simulink model "CDCJournalModel"  (R2017a)
settings: Solver=FixedStepAuto  StartTime=0.0  StopTime=p.T  FixedStep=0.001  RelTol=1e-3
StopFcn:
  | stopCallback
values from neighbouring files (symbols this model uses):
  p = simulationParametersClass    [preLoadCallback.m]
undefined symbols (not defined in the file or in its folder): rudderTable, wingTable
libraries: simulink x9, myLibrary x9, lowLevel x6, dspsigops x1
settings Model: Creator=M.Cobb  LastModifiedBy=M.Cobb
settings DataIOCC: SaveFormat=Structure

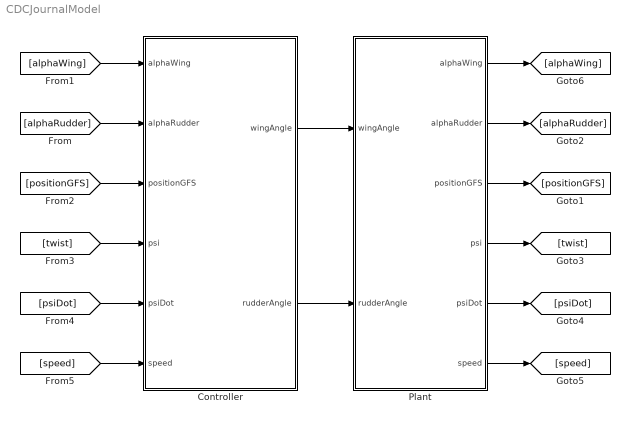
== system CDCJournalModel ==
  Controller : Subsystem
  Plant : Subsystem
  wires:
  Controller/1(wingAngle) -> Plant/1(wingAngle)
  Plant/1(alphaWing) -> [alphaWing]
  Plant/2(alphaRudder) -> [alphaRudder]
  [alphaWing] -> Controller/1(alphaWing)
  [alphaRudder] -> Controller/2(alphaRudder)
  Plant/3(positionGFS) -> [positionGFS]
  [positionGFS] -> Controller/3(positionGFS)
  Plant/4(psi) -> [twist]
  [twist] -> Controller/4("psi ")
  [psiDot] -> Controller/5(psiDot)
  [speed] -> Controller/6(speed)
  Plant/5(psiDot) -> [psiDot]
  Plant/6(speed) -> [speed]
  Controller/2(rudderAngle) -> Plant/2(rudderAngle)

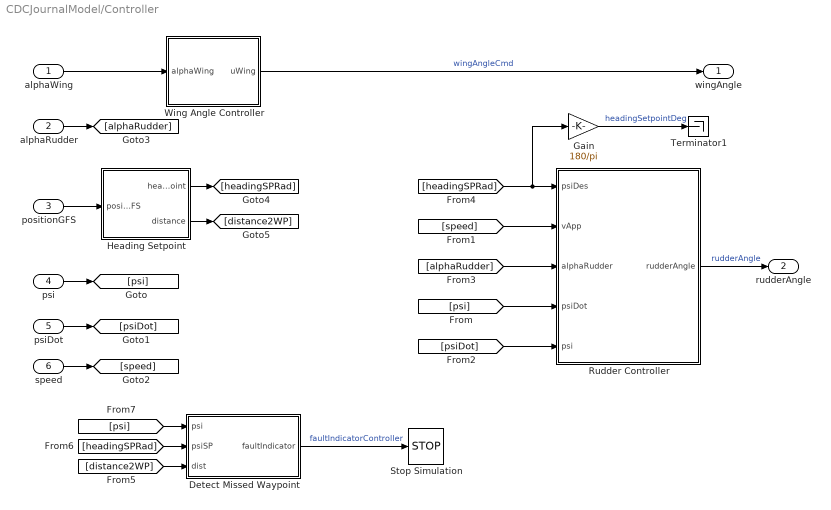
== system CDCJournalModel/Controller ==
  alphaWing : Inport
  alphaRudder : Inport  Port=2
  positionGFS : Inport  Port=3
  "psi " : Inport  Port=4
  psiDot : Inport  Port=5
  speed : Inport  Port=6
  Detect Missed Waypoint : Subsystem
  Gain : Gain  Gain=180/pi
  Heading Setpoint : Subsystem
  Rudder Controller : Subsystem
  Stop Simulation : Stop
  Terminator1 : Terminator
  Wing Angle Controller : Subsystem
  wingAngle : Outport
  rudderAngle : Outport  Port=2
  wires:
  alphaWing/1 -> Wing Angle Controller/1(alphaWing)
  Wing Angle Controller/1(uWing) -> wingAngle/1  "wingAngleCmd"
  positionGFS/1 -> Heading Setpoint/1(positionGFS)
  Heading Setpoint/1(headingSetpoint) -> [headingSPRad]
  "psi "/1 -> [psi]
  psiDot/1 -> [psiDot]
  speed/1 -> [speed]
  alphaRudder/1 -> [alphaRudder]
  Gain/1 -> Terminator1/1  "headingSetpointDeg"
  Rudder Controller/1(rudderAngle) -> rudderAngle/1  "rudderAngle"
  [speed] -> Rudder Controller/2(vApp)
  [headingSPRad] -> Gain/1, Rudder Controller/1(psiDes)
  [alphaRudder] -> Rudder Controller/3(alphaRudder)
  [psi] -> Rudder Controller/4(psiDot)
  [psiDot] -> Rudder Controller/5(psi)
  Heading Setpoint/2(distance) -> [distance2WP]
  [distance2WP] -> Detect Missed Waypoint/3("dist ")
  [psi] -> Detect Missed Waypoint/1(psi)
  [headingSPRad] -> Detect Missed Waypoint/2(psiSP)
  Detect Missed Waypoint/1(faultIndicator) -> Stop Simulation/1  "faultIndicatorController"

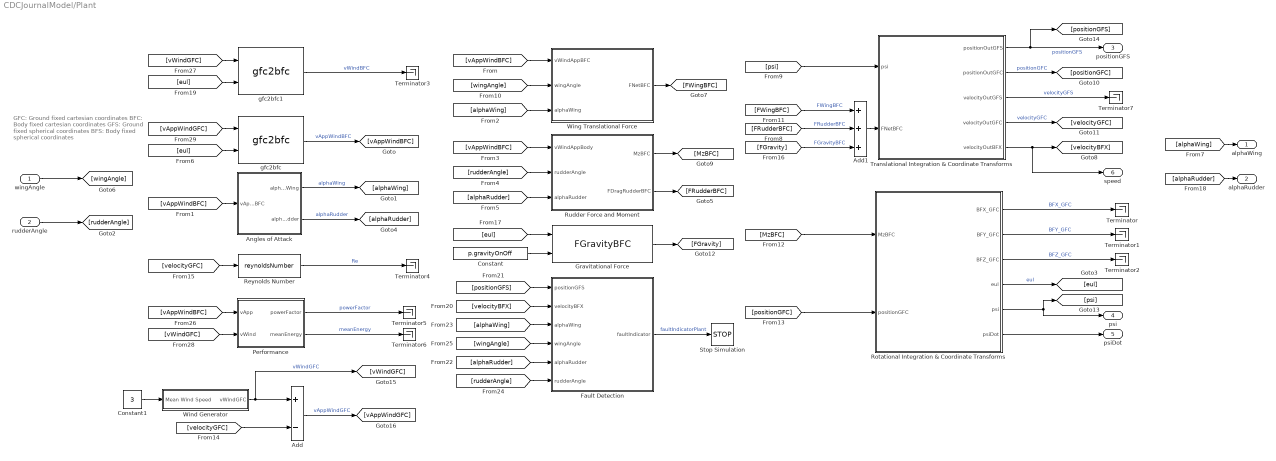
== system CDCJournalModel/Plant ==
  note: GFC: Ground fixed cartesian coordinates
      | BFC:  Body fixed cartesian coordinates
      | GFS: Ground fixed spherical coordinates
      | BFS: Body fixed spherical coordinates
  wingAngle : Inport
  rudderAngle : Inport  Port=2
  Add : Sum  Inputs=+-
  Add1 : Sum  Inputs=+++
  Angles of Attack : Subsystem
  Constant : Constant  Value=p.gravityOnOff
  Constant1 : Constant  Value=3
  Fault Detection : Subsystem
  Gravitational Force : myLibrary/FGravityBFC
  Performance : Subsystem
  Reynolds Number : myLibrary/reynoldsNumber
  Rotational Integration & Coordinate Transforms : Subsystem
  Rudder Force and Moment : Subsystem
  Stop Simulation : Stop
  Terminator{,1..7} (8 alike) : Terminator
  Translational Integration & Coordinate Transforms : Subsystem
  Wind Generator : Subsystem
  Wing Translational Force : Subsystem
  gfc2bfc : myLibrary/gfc2bfc
  gfc2bfc1 : myLibrary/gfc2bfc
  alphaWing : Outport
  alphaRudder : Outport  Port=2
  positionGFS : Outport  Port=3
  psi : Outport  Port=4
  psiDot : Outport  Port=5
  speed : Outport  Port=6
  wires:
  Wind Generator/1(vWindGFC) -> [vWindGFC], Add/1  "vWindGFC"
  [vAppWindBFC] -> Angles of Attack/1(vAppWindBFC)
  Angles of Attack/1(alphaWing) -> [alphaWing]  "alphaWing"
  [vAppWindBFC] -> Wing Translational Force/1(vWindAppBFC)
  Add/1 -> [vAppWindGFC]  "vAppWindGFC"
  [vAppWindBFC] -> Rudder Force and Moment/1(vWindAppBody)
  rudderAngle/1 -> [rudderAngle]
  [rudderAngle] -> Rudder Force and Moment/2(rudderAngle)
  Translational Integration & Coordinate Transforms/2(positionOutGFC) -> [positionGFC]  "positionGFC"
  Rudder Force and Moment/2(FDragRudderBFC) -> [FRudderBFC]
  [alphaWing] -> Wing Translational Force/3(alphaWing)
  [psi] -> Translational Integration & Coordinate Transforms/1(psi)
  Angles of Attack/2(alphaRudder) -> [alphaRudder]  "alphaRudder"
  [alphaRudder] -> Rudder Force and Moment/3(alphaRudder)
  wingAngle/1 -> [wingAngle]
  [FRudderBFC] -> Add1/2  "FRudderBFC"
  Wing Translational Force/1(FNetBFC) -> [FWingBFC]
  [wingAngle] -> Wing Translational Force/2(wingAngle)
  Add1/1 -> Translational Integration & Coordinate Transforms/2(FNetBFC)
  [FWingBFC] -> Add1/1  "FWingBFC"
  Rudder Force and Moment/1(MzBFC) -> [MzBFC]
  [MzBFC] -> Rotational Integration & Coordinate Transforms/1(MzBFC)
  [positionGFC] -> Rotational Integration & Coordinate Transforms/2(positionGFC)
  Rotational Integration & Coordinate Transforms/4(eul) -> [eul]  "eul"
  Rotational Integration & Coordinate Transforms/1(BFX_GFC) -> Terminator/1  "BFX_GFC"
  Rotational Integration & Coordinate Transforms/2(BFY_GFC) -> Terminator1/1  "BFY_GFC"
  Rotational Integration & Coordinate Transforms/3(BFZ_GFC) -> Terminator2/1  "BFZ_GFC"
  Translational Integration & Coordinate Transforms/4(velocityOutGFC) -> [velocityGFC]  "velocityGFC"
  [velocityGFC] -> Add/2
  [velocityGFC] -> Reynolds Number/1
  Reynolds Number/1 -> Terminator4/1  "Re"
  [FGravity] -> Add1/3  "FGravityBFC"
  Gravitational Force/1 -> [FGravity]
  [eul] -> Gravitational Force/1
  Translational Integration & Coordinate Transforms/1(positionOutGFS) -> positionGFS/1, [positionGFS]  "positionGFS"
  Translational Integration & Coordinate Transforms/3(velocityOutGFS) -> Terminator7/1  "velocityGFS"
  [eul] -> gfc2bfc1/2
  gfc2bfc1/1 -> Terminator3/1  "vWindBFC"
  Rotational Integration & Coordinate Transforms/5(psi) -> [psi], psi/1
  Constant/1 -> Gravitational Force/2
  [alphaWing] -> alphaWing/1
  [alphaRudder] -> alphaRudder/1
  Constant1/1 -> Wind Generator/1(Mean Wind Speed)
  Translational Integration & Coordinate Transforms/5(velocityOutBFX) -> speed/1, [velocityBFX]
  [velocityBFX] -> Fault Detection/2(velocityBFX)
  [positionGFS] -> Fault Detection/1(positionGFS)
  Fault Detection/1(faultIndicator) -> Stop Simulation/1  "faultIndicatorPlant"
  [alphaRudder] -> Fault Detection/5(alphaRudder)
  [alphaWing] -> Fault Detection/3(alphaWing)
  [rudderAngle] -> Fault Detection/6(rudderAngle)
  [wingAngle] -> Fault Detection/4(wingAngle)
  Rotational Integration & Coordinate Transforms/6(psiDot) -> psiDot/1
  [vWindGFC] -> gfc2bfc1/1
  [vAppWindBFC] -> Performance/1(vApp)
  [vWindGFC] -> Performance/2(vWind)
  gfc2bfc/1 -> [vAppWindBFC]  "vAppWindBFC"
  [eul] -> gfc2bfc/2
  [vAppWindGFC] -> gfc2bfc/1
  Performance/1(powerFactor) -> Terminator5/1  "powerFactor"
  Performance/2(meanEnergy) -> Terminator6/1  "meanEnergy"

== system CDCJournalModel/Controller/Detect Missed Waypoint ==
  psi : Inport
  psiSP : Inport  Port=2
  "dist " : Inport  Port=3
  Abs : Abs
  Add : Sum  Inputs=+-
  Add1 : Sum  Inputs=-+
  Compare To Constant : simulink/Logic and Bit Operations/Compare To Constant  relop=>=  const=pi/2  OutDataTypeStr=boolean
  Compare To Constant1 : simulink/Logic and Bit Operations/Compare To Constant  relop=<  const=0  OutDataTypeStr=boolean
  Delay : Delay  DelayLength=1  InitialCondition=0
  Logical Operator : Logic  AllPortsSameDT=off  OutDataTypeStr=boolean
  faultIndicator : Outport
  wires:
  Compare To Constant/1 -> Logical Operator/1
  psiSP/1 -> Add/1
  Delay/1 -> Add1/2
  Add1/1 -> Compare To Constant1/1
  Add/1 -> Abs/1
  psi/1 -> Add/2
  Logical Operator/1 -> faultIndicator/1  "faultMissedWaypoint"
  Compare To Constant1/1 -> Logical Operator/2
  Abs/1 -> Compare To Constant/1
  "dist "/1 -> Delay/1, Add1/1

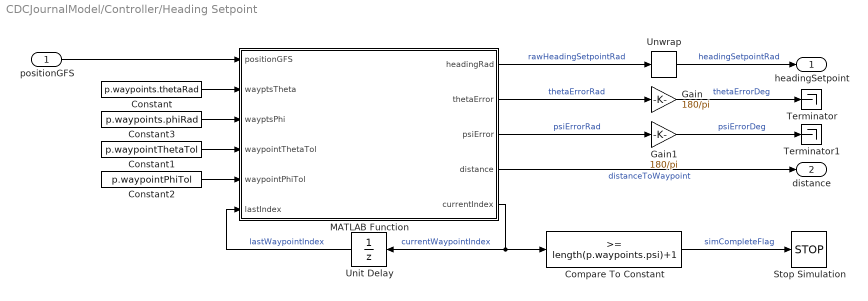
== system CDCJournalModel/Controller/Heading Setpoint ==
  positionGFS : Inport
  Compare To Constant : simulink/Logic and Bit Operations/Compare To Constant  relop=>=  const=length(p.waypoints.psi)+1  OutDataTypeStr=boolean
  Constant : Constant  Value=p.waypoints.thetaRad
  Constant1 : Constant  Value=p.waypointThetaTol
  Constant2 : Constant  Value=p.waypointPhiTol
  Constant3 : Constant  Value=p.waypoints.phiRad
  Gain : Gain  Gain=180/pi
  Gain1 : Gain  Gain=180/pi
  MATLAB Function : MATLAB Function  TreatAsAtomicUnit=on
  Stop Simulation : Stop
  Terminator : Terminator
  Terminator1 : Terminator
  Unit Delay : UnitDelay  InitialCondition=1  SampleTime=-1
  Unwrap : dspsigops/Unwrap  tol=pi  InputProcessing=Columns as channels (frame based)  running=off
  headingSetpoint : Outport
  distance : Outport  Port=2
  wires:
  Constant1/1 -> MATLAB Function/4(waypointThetaTol)
  Unit Delay/1 -> MATLAB Function/6(lastIndex)  "lastWaypointIndex"
  Constant2/1 -> MATLAB Function/5(waypointPhiTol)
  positionGFS/1 -> MATLAB Function/1(positionGFS)
  Constant/1 -> MATLAB Function/2(wayptsTheta)
  Constant3/1 -> MATLAB Function/3(wayptsPhi)
  MATLAB Function/2(thetaError) -> Gain/1  "thetaErrorRad"
  MATLAB Function/3(psiError) -> Gain1/1  "psiErrorRad"
  Gain/1 -> Terminator/1  "thetaErrorDeg"
  Gain1/1 -> Terminator1/1  "psiErrorDeg"
  MATLAB Function/5(currentIndex) -> Compare To Constant/1, Unit Delay/1  "currentWaypointIndex"
  MATLAB Function/1(headingRad) -> Unwrap/1  "rawHeadingSetpointRad"
  Unwrap/1 -> headingSetpoint/1  "headingSetpointRad"
  Compare To Constant/1 -> Stop Simulation/1  "simCompleteFlag"
  MATLAB Function/4(distance) -> distance/1  "distanceToWaypoint"

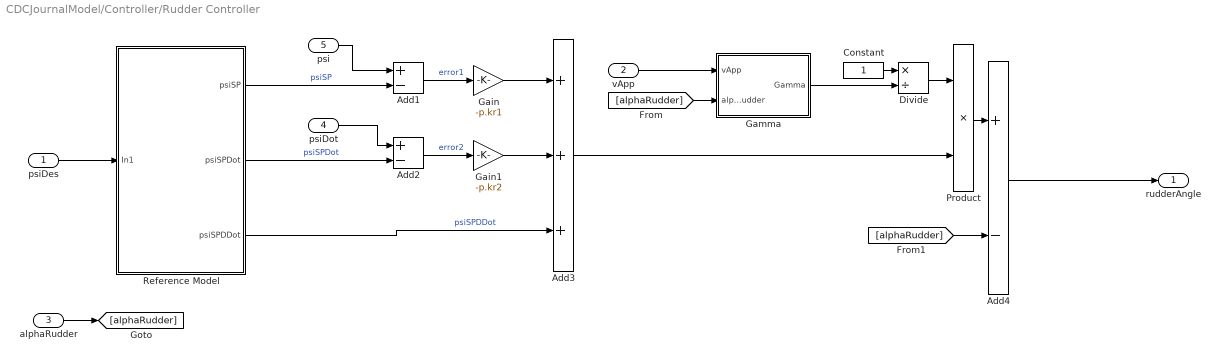
== system CDCJournalModel/Controller/Rudder Controller ==
  psiDes : Inport
  vApp : Inport  Port=2
  alphaRudder : Inport  Port=3
  psiDot : Inport  Port=4
  psi : Inport  Port=5
  Add1 : Sum  Inputs=+-
  Add2 : Sum  Inputs=+-
  Add3 : Sum  Inputs=+++
  Add4 : Sum  Inputs=+-
  Constant : Constant
  Divide : Product  Inputs=*/
  Gain : Gain  Gain=-p.kr1
  Gain1 : Gain  Gain=-p.kr2
  Gamma : Subsystem
  Product : Product
  Reference Model : Subsystem
  rudderAngle : Outport
  wires:
  alphaRudder/1 -> [alphaRudder]
  vApp/1 -> Gamma/1(vApp)
  [alphaRudder] -> Gamma/2(alphaRudder)
  [alphaRudder] -> Add4/2
  Product/1 -> Add4/1
  Gamma/1(Gamma) -> Divide/2
  Divide/1 -> Product/1
  Constant/1 -> Divide/1
  Add2/1 -> Gain1/1  "error2"
  Add1/1 -> Gain/1  "error1"
  Reference Model/1(psiSP) -> Add1/2  "psiSP"
  Reference Model/2(psiSPDot) -> Add2/2  "psiSPDot"
  psi/1 -> Add1/1
  Gain1/1 -> Add3/2
  psiDot/1 -> Add2/1
  Reference Model/3(psiSPDDot) -> Add3/3  "psiSPDDot"
  Gain/1 -> Add3/1
  psiDes/1 -> Reference Model/1(In1)
  Add3/1 -> Product/2
  Add4/1 -> rudderAngle/1

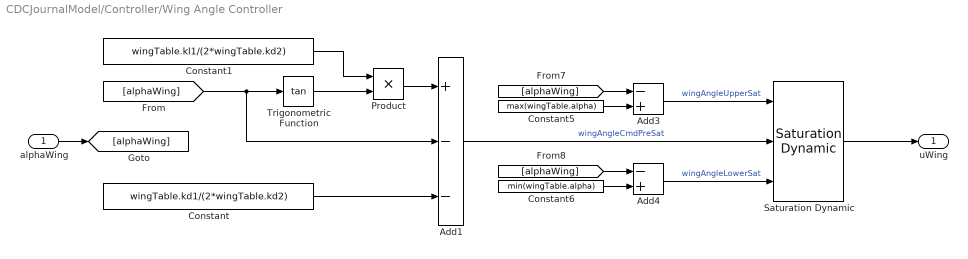
== system CDCJournalModel/Controller/Wing Angle Controller ==
  alphaWing : Inport
  Add1 : Sum  Inputs=+--
  Add3 : Sum  Inputs=-+
  Add4 : Sum  Inputs=-+
  Constant : Constant  Value=wingTable.kd1/(2*wingTable.kd2)
  Constant1 : Constant  Value=wingTable.kl1/(2*wingTable.kd2)
  Constant5 : Constant  Value=max(wingTable.alpha)
  Constant6 : Constant  Value=min(wingTable.alpha)
  Product : Product
  Saturation Dynamic : simulink/Discontinuities/Saturation Dynamic  OutMin=[]  OutMax=[]  OutDataTypeStr=Inherit: Same as second input  OutDataType=fixdt(1, 16)  OutScaling=2^-10  DoSatur=off
  Trigonometric Function : Trigonometry  Operator=tan
  uWing : Outport
  wires:
  Trigonometric Function/1 -> Product/2
  Constant/1 -> Add1/3
  Product/1 -> Add1/1
  Constant1/1 -> Product/1
  alphaWing/1 -> [alphaWing]
  [alphaWing] -> Add1/2, Trigonometric Function/1
  Add1/1 -> Saturation Dynamic/2  "wingAngleCmdPreSat"
  Saturation Dynamic/1 -> uWing/1
  [alphaWing] -> Add3/1
  Constant5/1 -> Add3/2
  Add3/1 -> Saturation Dynamic/1  "wingAngleUpperSat"
  Constant6/1 -> Add4/2
  [alphaWing] -> Add4/1
  Add4/1 -> Saturation Dynamic/3  "wingAngleLowerSat"

== system CDCJournalModel/Plant/Angles of Attack ==
  vAppWindBFC : Inport
  Atan1 : Trigonometry  Operator=atan2
  Atan2 : Trigonometry  Operator=atan2
  Demux : Demux  Outputs=3
  Demux1 : Demux  Outputs=3
  Gain2 : Gain  Gain=-1
  Gain3 : Gain  Gain=-1
  Terminator1 : Terminator
  Terminator2 : Terminator
  deadband : myLibrary/deadband
  deadband1 : myLibrary/deadband
  alphaWing : Outport
  alphaRudder : Outport  Port=2
  wires:
  vAppWindBFC/1 -> Gain2/1
  Demux/1 -> Atan2/2
  Atan2/1 -> Gain3/1
  Atan1/1 -> deadband/1
  Demux/3 -> Atan2/1
  Gain3/1 -> deadband1/1
  Demux/2 -> Terminator1/1
  Demux1/3 -> Terminator2/1
  Gain2/1 -> Demux1/1, Demux/1
  deadband/1 -> alphaRudder/1
  deadband1/1 -> alphaWing/1
  Demux1/1 -> Atan1/2
  Demux1/2 -> Atan1/1

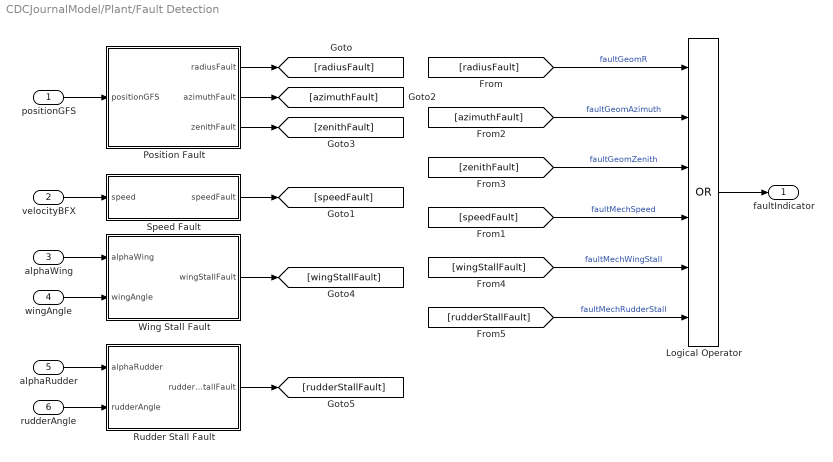
== system CDCJournalModel/Plant/Fault Detection ==
  positionGFS : Inport
  velocityBFX : Inport  Port=2
  alphaWing : Inport  Port=3
  wingAngle : Inport  Port=4
  alphaRudder : Inport  Port=5
  rudderAngle : Inport  Port=6
  Logical Operator : Logic  Operator=OR  Inputs=6  AllPortsSameDT=off  OutDataTypeStr=boolean
  Position Fault : Subsystem
  Rudder Stall Fault : Subsystem
  Speed Fault : Subsystem
  Wing Stall Fault : Subsystem
  faultIndicator : Outport
  wires:
  positionGFS/1 -> Position Fault/1(positionGFS)
  Logical Operator/1 -> faultIndicator/1
  Speed Fault/1(speedFault) -> [speedFault]
  velocityBFX/1 -> Speed Fault/1(speed)
  [radiusFault] -> Logical Operator/1  "faultGeomR"
  [speedFault] -> Logical Operator/4  "faultMechSpeed"
  [azimuthFault] -> Logical Operator/2  "faultGeomAzimuth"
  [zenithFault] -> Logical Operator/3  "faultGeomZenith"
  Wing Stall Fault/1(wingStallFault) -> [wingStallFault]
  alphaWing/1 -> Wing Stall Fault/1(alphaWing)
  alphaRudder/1 -> Rudder Stall Fault/1(alphaRudder)
  [wingStallFault] -> Logical Operator/5  "faultMechWingStall"
  [rudderStallFault] -> Logical Operator/6  "faultMechRudderStall"
  wingAngle/1 -> Wing Stall Fault/2(wingAngle)
  rudderAngle/1 -> Rudder Stall Fault/2(rudderAngle)
  Rudder Stall Fault/1(rudderStallFault) -> [rudderStallFault]
  Position Fault/1(radiusFault) -> [radiusFault]
  Position Fault/2(azimuthFault) -> [azimuthFault]
  Position Fault/3(zenithFault) -> [zenithFault]

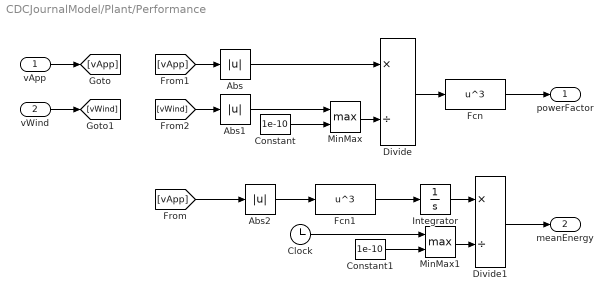
== system CDCJournalModel/Plant/Performance ==
  vApp : Inport
  vWind : Inport  Port=2
  Abs : Abs
  Abs1 : Abs
  Abs2 : Abs
  Clock : Clock
  Constant : Constant  Value=1e-10
  Constant1 : Constant  Value=1e-10
  Divide : Product  Inputs=*/
  Divide1 : Product  Inputs=*/
  Fcn : Fcn  Expr=u^3
  Fcn1 : Fcn  Expr=u^3
  Integrator : Integrator
  MinMax : MinMax  Function=max  Inputs=2
  MinMax1 : MinMax  Function=max  Inputs=2
  powerFactor : Outport
  meanEnergy : Outport  Port=2
  wires:
  Fcn/1 -> powerFactor/1
  Divide/1 -> Fcn/1
  Abs/1 -> Divide/1
  [vApp] -> Abs2/1
  Abs2/1 -> Fcn1/1
  Fcn1/1 -> Integrator/1
  Integrator/1 -> Divide1/1
  vApp/1 -> [vApp]
  vWind/1 -> [vWind]
  [vApp] -> Abs/1
  [vWind] -> Abs1/1
  Divide1/1 -> meanEnergy/1
  MinMax/1 -> Divide/2
  Abs1/1 -> MinMax/1
  Constant/1 -> MinMax/2
  Constant1/1 -> MinMax1/2
  MinMax1/1 -> Divide1/2
  Clock/1 -> MinMax1/1

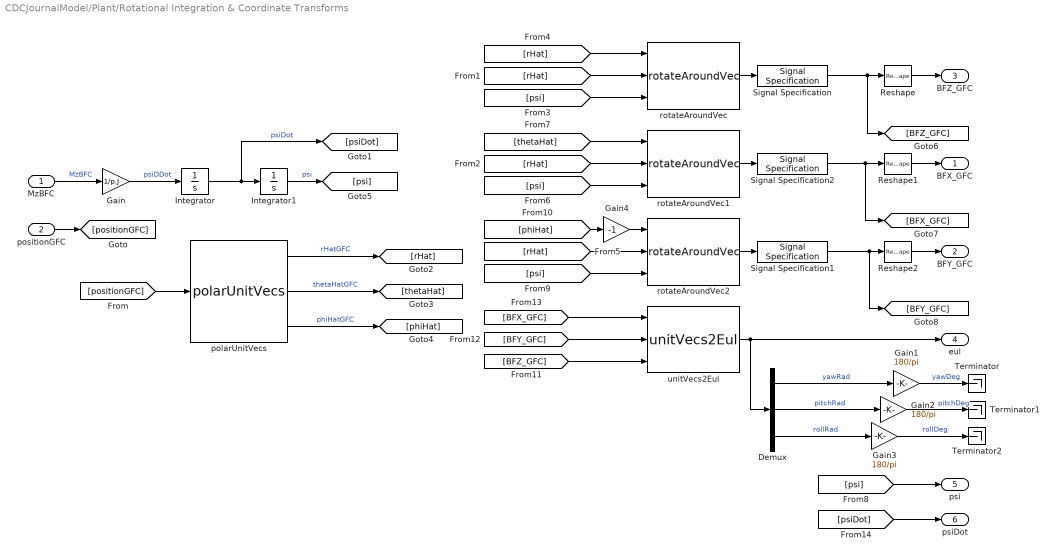
== system CDCJournalModel/Plant/Rotational Integration & Coordinate Transforms ==
  MzBFC : Inport  PortDimensions=1
  positionGFC : Inport  Port=2
  Demux : Demux  Outputs=3
  Gain : Gain  Gain=1/p.J
  Gain1 : Gain  Gain=180/pi
  Gain2 : Gain  Gain=180/pi
  Gain3 : Gain  Gain=180/pi
  Gain4 : Gain  Gain=-1
  Integrator : Integrator  InitialCondition=p.initOmega
  Integrator1 : Integrator  InitialCondition=p.initTwist
  Reshape : Reshape  OutputDimensions=[3 1]
  Reshape1 : Reshape  OutputDimensions=[3 1]
  Reshape2 : Reshape  OutputDimensions=[3 1]
  Signal Specification : SignalSpecification  Dimensions=[1 3]
  Signal Specification1 : SignalSpecification  Dimensions=[1 3]
  Signal Specification2 : SignalSpecification  Dimensions=[1 3]
  Terminator : Terminator
  Terminator1 : Terminator
  Terminator2 : Terminator
  polarUnitVecs : lowLevel/polarUnitVecs
  rotateAroundVec : lowLevel/rotateAroundVec
  rotateAroundVec1 : lowLevel/rotateAroundVec
  rotateAroundVec2 : lowLevel/rotateAroundVec
  unitVecs2Eul : myLibrary/unitVecs2Eul
  BFX_GFC : Outport
  BFY_GFC : Outport  Port=2
  BFZ_GFC : Outport  Port=3
  eul : Outport  Port=4  PortDimensions=3
  psi : Outport  Port=5  PortDimensions=1
  psiDot : Outport  Port=6  PortDimensions=1
  wires:
  MzBFC/1 -> Gain/1  "MzBFC"
  Integrator/1 -> [psiDot], Integrator1/1  "psiDot"
  Gain/1 -> Integrator/1  "psiDDot"
  positionGFC/1 -> [positionGFC]
  [positionGFC] -> polarUnitVecs/1
  polarUnitVecs/1 -> [rHat]  "rHatGFC"
  polarUnitVecs/2 -> [thetaHat]  "thetaHatGFC"
  polarUnitVecs/3 -> [phiHat]  "phiHatGFC"
  Integrator1/1 -> [psi]  "psi"
  [psi] -> rotateAroundVec/3
  [rHat] -> rotateAroundVec/1
  [rHat] -> rotateAroundVec/2
  [thetaHat] -> rotateAroundVec1/1
  [psi] -> rotateAroundVec1/3
  [rHat] -> rotateAroundVec1/2
  [phiHat] -> Gain4/1
  [psi] -> rotateAroundVec2/3
  [rHat] -> rotateAroundVec2/2
  unitVecs2Eul/1 -> Demux/1, eul/1
  [BFZ_GFC] -> unitVecs2Eul/3
  [BFY_GFC] -> unitVecs2Eul/2
  [BFX_GFC] -> unitVecs2Eul/1
  Demux/3 -> Gain3/1  "rollRad"
  Demux/2 -> Gain2/1  "pitchRad"
  Demux/1 -> Gain1/1  "yawRad"
  Gain1/1 -> Terminator/1  "yawDeg"
  Gain2/1 -> Terminator1/1  "pitchDeg"
  Gain3/1 -> Terminator2/1  "rollDeg"
  Gain4/1 -> rotateAroundVec2/1
  rotateAroundVec/1 -> Signal Specification/1
  rotateAroundVec1/1 -> Signal Specification2/1
  rotateAroundVec2/1 -> Signal Specification1/1
  Signal Specification/1 -> Reshape/1, [BFZ_GFC]
  Signal Specification2/1 -> [BFX_GFC], Reshape1/1
  Signal Specification1/1 -> [BFY_GFC], Reshape2/1
  Reshape/1 -> BFZ_GFC/1
  Reshape1/1 -> BFX_GFC/1
  Reshape2/1 -> BFY_GFC/1
  [psi] -> psi/1
  [psiDot] -> psiDot/1

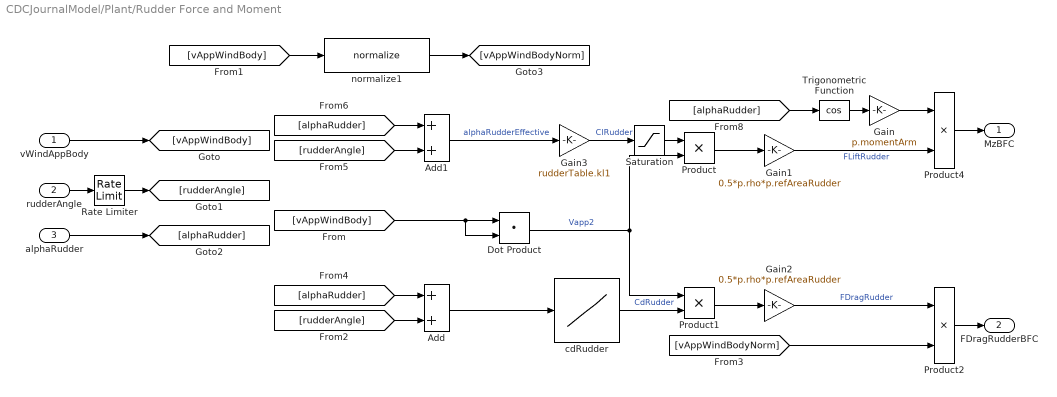
== system CDCJournalModel/Plant/Rudder Force and Moment ==
  vWindAppBody : Inport
  rudderAngle : Inport  Port=2
  alphaRudder : Inport  Port=3
  Add : Sum
  Add1 : Sum
  Dot Product : DotProduct  InputSameDT=on  OutDataTypeStr=Inherit: Inherit via internal rule
  Gain : Gain  Gain=p.momentArm
  Gain1 : Gain  Gain=0.5*p.rho*p.refAreaRudder
  Gain2 : Gain  Gain=0.5*p.rho*p.refAreaRudder
  Gain3 : Gain  Gain=rudderTable.kl1
  Product{,1..2,4} (4 alike) : Product
  Rate Limiter : RateLimiter  RisingSlewLimit=p.rudderAngleRateLimit*pi/180  FallingSlewLimit=-p.rudderAngleRateLimit*pi/180  SampleTimeMode=inherited
  Saturation : Saturate  UpperLimit=max(rudderTable.cl)  LowerLimit=min(rudderTable.cl)
  Trigonometric Function : Trigonometry  Operator=cos
  cdRudder : Lookup_n-D  NumberOfTableDimensions=1  BreakpointsForDimension1=rudderTable.alpha  Table=rudderTable.cd  InternalRulePriority=Speed  RndMeth=Simplest  InputSameDT=on
  normalize1 : myLibrary/normalize
  MzBFC : Outport
  FDragRudderBFC : Outport  Port=2
  wires:
  Gain3/1 -> Saturation/1  "ClRudder"
  [vAppWindBody] -> Dot Product/2, Dot Product/1
  Dot Product/1 -> Product1/1, Product/2  "Vapp2"
  vWindAppBody/1 -> [vAppWindBody]
  rudderAngle/1 -> Rate Limiter/1
  Product/1 -> Gain1/1
  cdRudder/1 -> Product1/2  "CdRudder"
  Product1/1 -> Gain2/1
  Gain2/1 -> Product2/1  "FDragRudder"
  [vAppWindBodyNorm] -> Product2/2
  alphaRudder/1 -> [alphaRudder]
  [rudderAngle] -> Add/2
  [alphaRudder] -> Add/1
  Add/1 -> cdRudder/1
  [rudderAngle] -> Add1/2
  [alphaRudder] -> Add1/1
  Add1/1 -> Gain3/1  "alphaRudderEffective"
  Gain1/1 -> Product4/2  "FLiftRudder"
  [vAppWindBody] -> normalize1/1
  normalize1/1 -> [vAppWindBodyNorm]
  Product2/1 -> FDragRudderBFC/1
  [alphaRudder] -> Trigonometric Function/1
  Product4/1 -> MzBFC/1
  Trigonometric Function/1 -> Gain/1
  Gain/1 -> Product4/1
  Saturation/1 -> Product/1
  Rate Limiter/1 -> [rudderAngle]

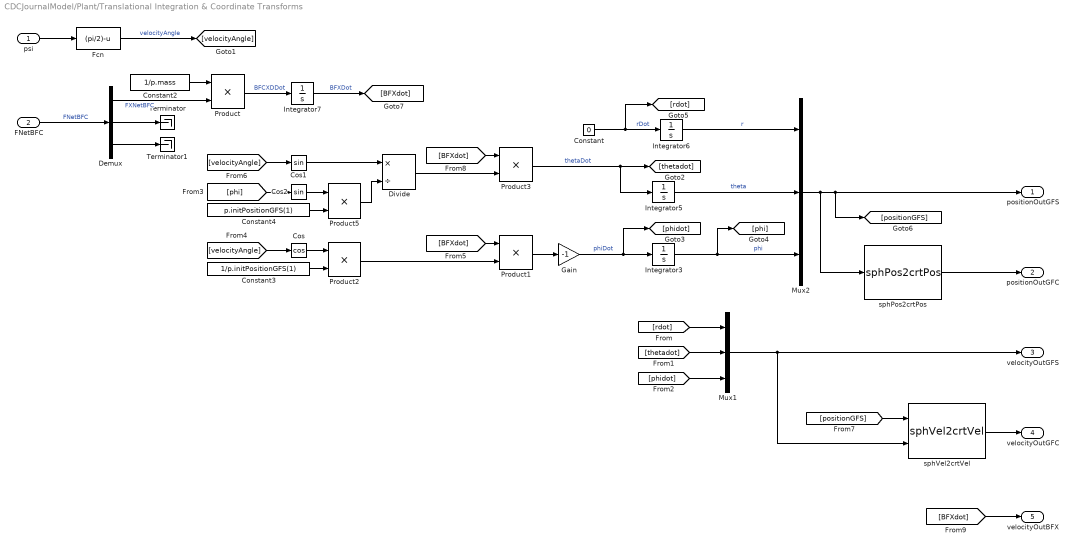
== system CDCJournalModel/Plant/Translational Integration & Coordinate Transforms ==
  psi : Inport
  FNetBFC : Inport  Port=2
  Constant : Constant  Value=0
  Constant2 : Constant  Value=1/p.mass
  Constant3 : Constant  Value=1/p.initPositionGFS(1)
  Constant4 : Constant  Value=p.initPositionGFS(1)
  Cos : Trigonometry  Operator=cos
  Cos1 : Trigonometry
  Cos2 : Trigonometry
  Demux : Demux  Outputs=3
  Divide : Product  Inputs=*/
  Fcn : Fcn  Expr=(pi/2)-u
  Gain : Gain  Gain=-1
  Integrator3 : Integrator  InitialCondition=p.initPositionGFS(3)
  Integrator5 : Integrator  InitialCondition=p.initPositionGFS(2)
  Integrator6 : Integrator  InitialCondition=p.initPositionGFS(1)
  Integrator7 : Integrator  InitialCondition=p.initVelocity
  Mux1 : Mux  Inputs=3
  Mux2 : Mux  Inputs=3
  Product{,1..3,5} (5 alike) : Product
  Terminator : Terminator
  Terminator1 : Terminator
  sphPos2crtPos : lowLevel/sphPos2crtPos
  sphVel2crtVel : lowLevel/sphVel2crtVel
  positionOutGFS : Outport  PortDimensions=3
  positionOutGFC : Outport  Port=2  PortDimensions=3
  velocityOutGFS : Outport  Port=3  PortDimensions=3
  velocityOutGFC : Outport  Port=4  PortDimensions=3
  velocityOutBFX : Outport  Port=5
  wires:
  Gain/1 -> [phidot], Integrator3/1  "phiDot"
  Integrator5/1 -> Mux2/2  "theta"
  Product3/1 -> Integrator5/1, [thetadot]  "thetaDot"
  Integrator3/1 -> [phi], Mux2/3  "phi"
  sphPos2crtPos/1 -> positionOutGFC/1
  sphVel2crtVel/1 -> velocityOutGFC/1
  [rdot] -> Mux1/1
  [thetadot] -> Mux1/2
  [phidot] -> Mux1/3
  FNetBFC/1 -> Demux/1  "FNetBFC"
  psi/1 -> Fcn/1
  Demux/1 -> Product/2  "FXNetBFC"
  Integrator6/1 -> Mux2/1  "r"
  Mux1/1 -> sphVel2crtVel/2, velocityOutGFS/1
  Constant/1 -> [rdot], Integrator6/1  "rDot"
  Mux2/1 -> sphPos2crtPos/1, [positionGFS], positionOutGFS/1
  [positionGFS] -> sphVel2crtVel/1
  Demux/2 -> Terminator/1
  Demux/3 -> Terminator1/1
  Constant2/1 -> Product/1
  Fcn/1 -> [velocityAngle]  "velocityAngle"
  [BFXdot] -> Product3/1
  [velocityAngle] -> Cos1/1
  Divide/1 -> Product3/2
  Cos1/1 -> Divide/1
  Constant4/1 -> Product5/2
  [phi] -> Cos2/1
  Cos2/1 -> Product5/1
  Product5/1 -> Divide/2
  [BFXdot] -> Product1/1
  [velocityAngle] -> Cos/1
  Product2/1 -> Product1/2
  Cos/1 -> Product2/1
  Constant3/1 -> Product2/2
  Product1/1 -> Gain/1
  Integrator7/1 -> [BFXdot]  "BFXDot"
  Product/1 -> Integrator7/1  "BFCXDDot"
  [BFXdot] -> velocityOutBFX/1

== system CDCJournalModel/Plant/Wind Generator ==
  Mean Wind Speed : Inport  Unit=m/s
  Constant : Constant  Value=0
  Constant1 : Constant  Value=0
  Mux : Mux  Inputs=3
  vWindGFC : Outport
  wires:
  Mean Wind Speed/1 -> Mux/1
  Constant1/1 -> Mux/2
  Constant/1 -> Mux/3
  Mux/1 -> [groundCartesian]
  [groundCartesian] -> vWindGFC/1

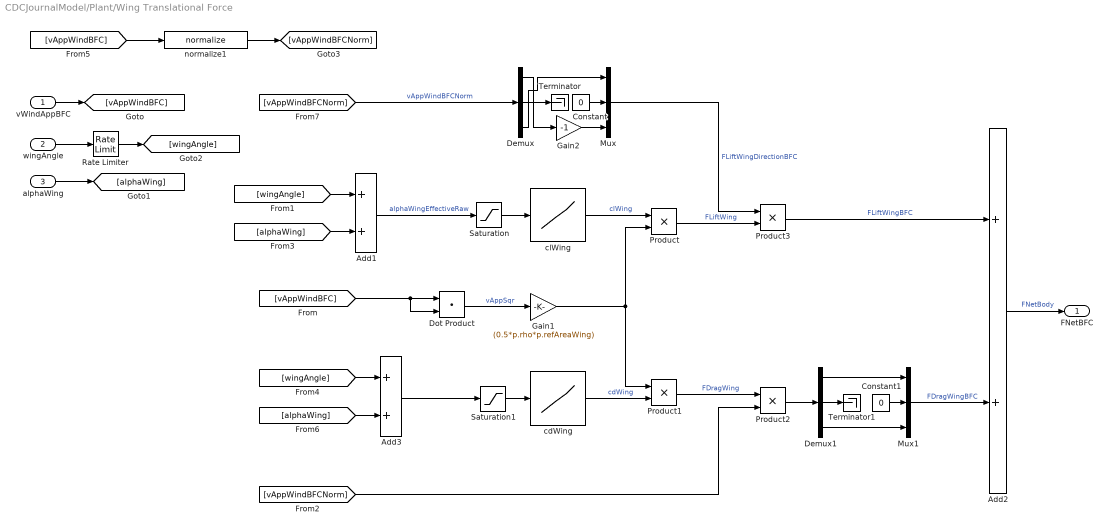
== system CDCJournalModel/Plant/Wing Translational Force ==
  vWindAppBFC : Inport
  wingAngle : Inport  Port=2
  alphaWing : Inport  Port=3
  Add1 : Sum
  Add2 : Sum
  Add3 : Sum
  Constant : Constant  Value=0
  Constant1 : Constant  Value=0
  Demux : Demux  Outputs=3
  Demux1 : Demux  Outputs=3
  Dot Product : DotProduct  InputSameDT=on  OutDataTypeStr=Inherit: Inherit via internal rule
  Gain1 : Gain  Gain=(0.5*p.rho*p.refAreaWing)
  Gain2 : Gain  Gain=-1
  Mux : Mux  Inputs=3
  Mux1 : Mux  Inputs=3
  Product{,1..3} (4 alike) : Product
  Rate Limiter : RateLimiter  RisingSlewLimit=p.wingAngleRateLimit*pi/180  FallingSlewLimit=-p.wingAngleRateLimit*pi/180  SampleTimeMode=inherited
  Saturation : Saturate  UpperLimit=max(wingTable.alpha)  LowerLimit=min(wingTable.alpha)
  Saturation1 : Saturate  UpperLimit=max(wingTable.alpha)  LowerLimit=min(wingTable.alpha)
  Terminator : Terminator
  Terminator1 : Terminator
  cdWing : Lookup_n-D  NumberOfTableDimensions=1  BreakpointsForDimension1=wingTable.alpha  Table=wingTable.cd  InternalRulePriority=Speed  RndMeth=Simplest  InputSameDT=on
  clWing : Lookup_n-D  NumberOfTableDimensions=1  BreakpointsForDimension1=wingTable.alpha  Table=wingTable.cl  InternalRulePriority=Speed  RndMeth=Simplest  InputSameDT=on
  normalize1 : myLibrary/normalize
  FNetBFC : Outport
  wires:
  Product1/1 -> Product2/1  "FDragWing"
  Mux1/1 -> Add2/2  "FDragWingBFC"
  Product/1 -> Product3/2  "FLiftWing"
  Product3/1 -> Add2/1  "FLiftWingBFC"
  Dot Product/1 -> Gain1/1  "vAppSqr"
  clWing/1 -> Product/1  "clWing"
  [vAppWindBFC] -> Dot Product/2, Dot Product/1
  Gain1/1 -> Product/2, Product1/1
  cdWing/1 -> Product1/2  "cdWing"
  vWindAppBFC/1 -> [vAppWindBFC]
  Add2/1 -> FNetBFC/1  "FNetBody"
  alphaWing/1 -> [alphaWing]
  wingAngle/1 -> Rate Limiter/1
  Add3/1 -> Saturation1/1
  [wingAngle] -> Add3/1
  [alphaWing] -> Add3/2
  Demux/2 -> Terminator/1
  Constant/1 -> Mux/2
  Demux/1 -> Gain2/1
  Mux/1 -> Product3/1  "FLiftWingDirectionBFC"
  Demux/3 -> Mux/1
  [vAppWindBFC] -> normalize1/1
  normalize1/1 -> [vAppWindBFCNorm]
  [vAppWindBFCNorm] -> Demux/1  "vAppWindBFCNorm"
  [vAppWindBFCNorm] -> Product2/2
  Gain2/1 -> Mux/3
  Demux1/2 -> Terminator1/1
  Constant1/1 -> Mux1/2
  Demux1/1 -> Mux1/1
  Product2/1 -> Demux1/1
  Demux1/3 -> Mux1/3
  Saturation/1 -> clWing/1
  Saturation1/1 -> cdWing/1
  [wingAngle] -> Add1/1
  [alphaWing] -> Add1/2
  Add1/1 -> Saturation/1  "alphaWingEffectiveRaw"
  Rate Limiter/1 -> [wingAngle]

== system CDCJournalModel/Controller/Rudder Controller/Gamma ==
  vApp : Inport
  alphaRudder : Inport  Port=2
  Constant : Constant  Value=1/2
  Constant1 : Constant  Value=p.rho
  Constant2 : Constant  Value=rudderTable.kl1
  Constant3 : Constant  Value=p.momentArm
  Constant4 : Constant  Value=1/p.J
  Constant5 : Constant  Value=p.refAreaRudder
  Product : Product  Inputs=8
  Product1 : Product
  Trigonometric Function : Trigonometry  Operator=cos
  Gamma : Outport
  wires:
  Constant4/1 -> Product/2
  Constant3/1 -> Product/7
  Constant5/1 -> Product/5
  Constant/1 -> Product/1
  Constant2/1 -> Product/6
  Constant1/1 -> Product/3
  Product1/1 -> Product/4
  vApp/1 -> Product1/2, Product1/1
  alphaRudder/1 -> Trigonometric Function/1
  Trigonometric Function/1 -> Product/8
  Product/1 -> Gamma/1

== system CDCJournalModel/Controller/Rudder Controller/Reference Model ==
  note: Reference Model:
      | 1/(tauR*s+1)^2
  In1 : Inport
  Add1 : Sum  Inputs=--+
  Gain : Gain  Gain=1/(p.tauR^2)
  Gain1 : Gain  Gain=2*p.tauR
  Integrator : Integrator
  Integrator2 : Integrator
  psiSP : Outport
  psiSPDot : Outport  Port=2
  psiSPDDot : Outport  Port=3
  wires:
  Gain/1 -> psiSPDDot/1, Integrator/1  "psiSPDDot"
  Integrator/1 -> psiSPDot/1, Gain1/1, Integrator2/1  "psiSPDot"
  Add1/1 -> Gain/1
  Integrator2/1 -> Add1/2, psiSP/1  "psiSP"
  In1/1 -> Add1/3  "psiDes"
  Gain1/1 -> Add1/1

== system CDCJournalModel/Plant/Fault Detection/Position Fault ==
  positionGFS : Inport
  Azimuth Fault : Subsystem
  Constant1 : Constant  Value=0
  Constant2 : Constant
  Constant3 : Constant
  Demux : Demux  Outputs=3
  Product : Product
  Product1 : Product
  Product2 : Product
  Radius Fault : Subsystem
  Zenith Fault : Subsystem
  radiusFault : Outport
  azimuthFault : Outport  Port=2
  zenithFault : Outport  Port=3
  wires:
  positionGFS/1 -> Demux/1
  Demux/1 -> Radius Fault/1(r)
  Radius Fault/1(fault) -> Product2/2
  Azimuth Fault/1(fault) -> Product1/2
  Zenith Fault/1(fault) -> Product/2
  Demux/2 -> Azimuth Fault/1(theta)
  Demux/3 -> Zenith Fault/1(phi)
  Product/1 -> zenithFault/1
  Product1/1 -> azimuthFault/1
  Product2/1 -> radiusFault/1
  Constant3/1 -> Product/1
  Constant1/1 -> Product1/1
  Constant2/1 -> Product2/1

== system CDCJournalModel/Plant/Fault Detection/Rudder Stall Fault ==
  alphaRudder : Inport
  rudderAngle : Inport  Port=2
  Add : Sum
  Compare : RelationalOperator  Operator=<=  OutDataTypeStr=boolean  RndMeth=Nearest  InputSameDT=on
  Compare1 : RelationalOperator  OutDataTypeStr=boolean  RndMeth=Nearest  InputSameDT=on
  Constant : Constant  Value=min(rudderTable.alpha)
  Constant1 : Constant  Value=max(rudderTable.alpha)
  Constant3 : Constant  Value=0
  Logical Operator : Logic  Operator=OR  AllPortsSameDT=off  OutDataTypeStr=boolean
  Product : Product
  rudderStallFault : Outport
  wires:
  Compare1/1 -> Logical Operator/2
  Constant1/1 -> Compare1/1
  Constant/1 -> Compare/1
  Compare/1 -> Logical Operator/1
  rudderAngle/1 -> Add/2
  alphaRudder/1 -> Add/1
  Add/1 -> Compare1/2, Compare/2
  Constant3/1 -> Product/1
  Logical Operator/1 -> Product/2
  Product/1 -> rudderStallFault/1

== system CDCJournalModel/Plant/Fault Detection/Speed Fault ==
  note: If body fixed speed in x is negative
  speed : Inport
  Compare To Constant : simulink/Logic and Bit Operations/Compare To Constant  relop=<=  const=0  OutDataTypeStr=boolean
  Constant3 : Constant
  Product : Product
  speedFault : Outport
  wires:
  speed/1 -> Compare To Constant/1
  Compare To Constant/1 -> Product/2
  Product/1 -> speedFault/1
  Constant3/1 -> Product/1

== system CDCJournalModel/Plant/Fault Detection/Wing Stall Fault ==
  alphaWing : Inport
  wingAngle : Inport  Port=2
  Add : Sum
  Compare : RelationalOperator  Operator=>  OutDataTypeStr=boolean  RndMeth=Nearest  InputSameDT=on
  Compare1 : RelationalOperator  Operator=<  OutDataTypeStr=boolean  RndMeth=Nearest  InputSameDT=on
  Constant : Constant  Value=min(wingTable.alpha)
  Constant1 : Constant  Value=max(wingTable.alpha)
  Constant3 : Constant
  Logical Operator : Logic  Operator=OR  AllPortsSameDT=off  OutDataTypeStr=boolean
  Product : Product
  wingStallFault : Outport
  wires:
  Compare/1 -> Logical Operator/1
  Compare1/1 -> Logical Operator/2
  Constant/1 -> Compare/1
  Constant1/1 -> Compare1/1
  alphaWing/1 -> Add/1
  wingAngle/1 -> Add/2
  Add/1 -> Compare1/2, Compare/2
  Logical Operator/1 -> Product/2
  Product/1 -> wingStallFault/1
  Constant3/1 -> Product/1

== system CDCJournalModel/Plant/Fault Detection/Position Fault/Azimuth Fault ==
  note: If azimuth exceeds +/- ? deg
  theta : Inport
  Abs : Abs
  Compare To Constant : simulink/Logic and Bit Operations/Compare To Constant  relop=>=  const=(180*pi/180)  OutDataTypeStr=boolean
  fault : Outport
  wires:
  Compare To Constant/1 -> fault/1
  Abs/1 -> Compare To Constant/1
  theta/1 -> Abs/1

== system CDCJournalModel/Plant/Fault Detection/Position Fault/Radius Fault ==
  r : Inport
  Abs : Abs
  Add : Sum  Inputs=+-
  Compare To Constant : simulink/Logic and Bit Operations/Compare To Constant  relop=>=  const=0.01  OutDataTypeStr=boolean
  Divide : Product  Inputs=*/
  r Target : Constant  Value=p.initPositionGFS(1)
  fault : Outport
  wires:
  r Target/1 -> Divide/2, Add/2
  Add/1 -> Abs/1
  Compare To Constant/1 -> fault/1
  r/1 -> Add/1
  Abs/1 -> Divide/1
  Divide/1 -> Compare To Constant/1

== system CDCJournalModel/Plant/Fault Detection/Position Fault/Zenith Fault ==
  note: If zenith drops below 10 deg or goes above 80 deg.
  phi : Inport
  Abs : Abs
  Compare To Constant : simulink/Logic and Bit Operations/Compare To Constant  relop=<=  const=(10*pi/180)  OutDataTypeStr=boolean
  Compare To Constant1 : simulink/Logic and Bit Operations/Compare To Constant  relop=>=  const=(80*pi/180)  OutDataTypeStr=boolean
  Logical Operator : Logic  Operator=OR  AllPortsSameDT=off  OutDataTypeStr=boolean
  fault : Outport
  wires:
  Logical Operator/1 -> fault/1
  Abs/1 -> Compare To Constant1/1, Compare To Constant/1
  phi/1 -> Abs/1
  Compare To Constant/1 -> Logical Operator/1
  Compare To Constant1/1 -> Logical Operator/2

== matlab function CDCJournalModel/Controller/Heading Setpoint/MATLAB Function ==
  data: positionGFS input; headingRad output; thetaError output; psiError output; distance output; wayptsTheta input; wayptsPhi input; waypointThetaTol input; waypointPhiTol input; lastIndex input; currentIndex output
function [headingRad,thetaError,psiError,distance,currentIndex] = ...
    calculateHeading(positionGFS,wayptsTheta,wayptsPhi,waypointThetaTol,waypointPhiTol,lastIndex)

currentIndex = lastIndex;

while currentIndex <= length(wayptsTheta) &&...
        abs(positionGFS(2)-wayptsTheta(currentIndex))<=waypointThetaTol &&...
        abs(positionGFS(3)-wayptsPhi(currentIndex))<=waypointPhiTol
        
    currentIndex = currentIndex +1;
end

if currentIndex <= length(wayptsTheta)
    lat1 = (pi/2)-positionGFS(3);
    lon1 = positionGFS(2);
    lat2 = (pi/2)-wayptsPhi(currentIndex);
    lon2 = wayptsTheta(currentIndex);
    % Inputs LAT1, LON1, LAT2, LON2 are in units of radians.
    
    headingRad = (pi/2) - atan2(cos(lat2) .* sin(lon2-lon1),...
        cos(lat1) .* sin(lat2) - sin(lat1) .* cos(lat2) .* cos(lon2-lon1));
    
    % Azimuths are undefined at the poles, so we choose a convention: zero at
    % the north pole and pi at the south pole.
    headingRad(lat1 <= -pi/2) = 0;
    headingRad(lat2 >=  pi/2) = 0;
    headingRad(lat2 <= -pi/2) = pi;
    headingRad(lat1 >=  pi/2) = pi;
    % if currentIndex ==2
    %     1+1;
    % end
    
    thetaError = wayptsTheta(currentIndex)-positionGFS(2);
    psiError   = wayptsPhi(currentIndex)-positionGFS(3);
else
    lat1 = (pi/2)-positionGFS(3);
    lon1 = positionGFS(2);
    lat2 = (pi/2)-wayptsPhi(currentIndex-1);
    lon2 = wayptsTheta(currentIndex-1);
    % Inputs LAT1, LON1, LAT2, LON2 are in units of radians.
    
    headingRad = (pi/2) - atan2(cos(lat2) .* sin(lon2-lon1),...
        cos(lat1) .* sin(lat2) - sin(lat1) .* cos(lat2) .* cos(lon2-lon1));
    
    % Azimuths are undefined at the poles, so we choose a convention: zero at
    % the north pole and pi at the south pole.
    headingRad(lat1 <= -pi/2) = 0;
    headingRad(lat2 >=  pi/2) = 0;
    headingRad(lat2 <= -pi/2) = pi;
    headingRad(lat1 >=  pi/2) = pi;
    % if currentIndex ==2
    %     1+1;
    % end
    
    thetaError = wayptsTheta(currentIndex-1)-positionGFS(2);
    psiError   = wayptsPhi(currentIndex-1)-positionGFS(3);
    
end

% Calculate great circle distance between points on a sphere using the
% Haversine Formula.  LAT1, LON1, LAT2, and LON2 are in radians.  RNG is a
% length and has the same units as the radius of the sphere, R.  (If R is
% 1, then RNG is effectively arc length in radians.)

a = sin((lat2-lat1)/2).^2 + cos(lat1) .* cos(lat2) .* sin((lon2-lon1)/2).^2;

% Ensure that a falls in the closed interval [0 1].
a(a < 0) = 0;
a(a > 1) = 1;

distance = positionGFS(1) * 2 * atan2(sqrt(a),sqrt(1 - a));

end
